simulink library "flowSpeedCtrl"  (R2020a)
settings: Solver=VariableStepAuto  StartTime=0.0  StopTime=10.0  RelTol=1e-3
settings Model: Creator=Ayaz  LastModifiedBy=Ayaz

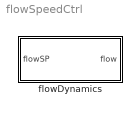
== system flowSpeedCtrl ==
  flowDynamics : Subsystem

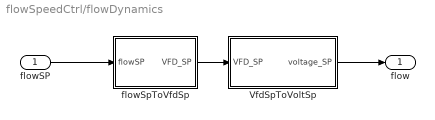
== system flowSpeedCtrl/flowDynamics ==
  flowSP : Inport
  VfdSpToVoltSp : Subsystem
  flowSpToVfdSp : Subsystem
  flow : Outport
  wires:
  flowSP/1 -> flowSpToVfdSp/1(flowSP)
  flowSpToVfdSp/1(VFD_SP) -> VfdSpToVoltSp/1(VFD_SP)
  VfdSpToVoltSp/1(voltage_SP) -> flow/1

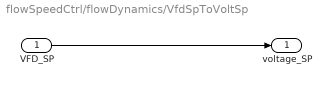
== system flowSpeedCtrl/flowDynamics/VfdSpToVoltSp ==
  VFD_SP : Inport
  voltage_SP : Outport
  wires:
  VFD_SP/1 -> voltage_SP/1

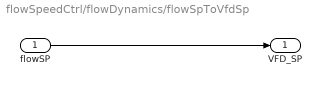
== system flowSpeedCtrl/flowDynamics/flowSpToVfdSp ==
  flowSP : Inport
  VFD_SP : Outport
  wires:
  flowSP/1 -> VFD_SP/1
